simulink model "Drone_human_obstacle"  (R2024a)
settings: Solver=VariableStepAuto  StartTime=0.0  StopTime=10.0  RelTol=1e-3
undefined symbols (not defined in the file or in its folder): Angle, Axis, gray
libraries: eeGeneralControl x2, robotcorelib x1
settings Model: Creator=quentinlandon  LastModifiedBy=quentinlandon

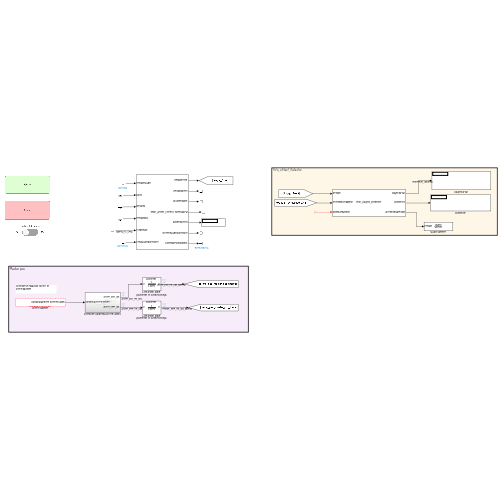
[thumbnail: Simulink's stored preview of the top-level diagram]
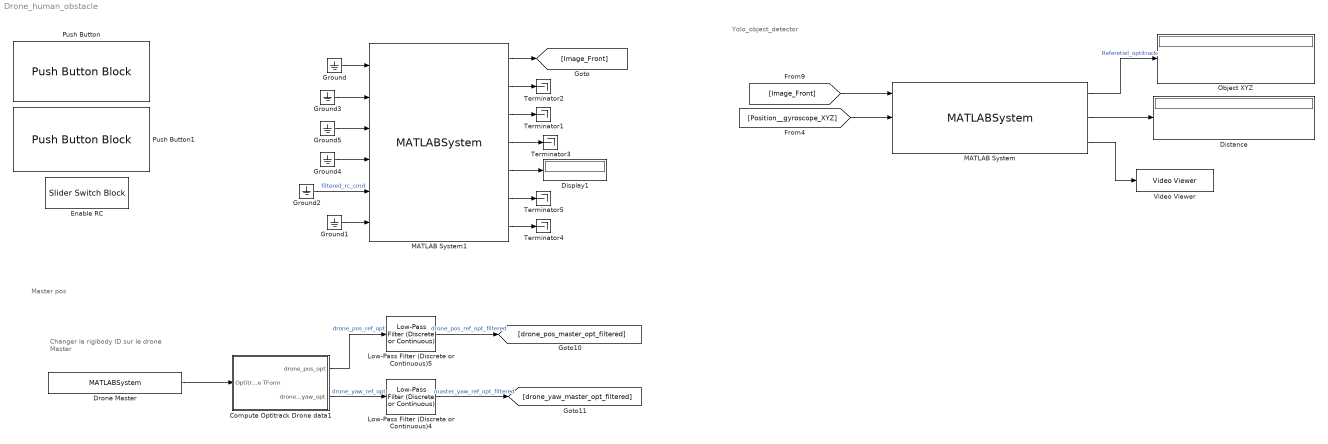
== system Drone_human_obstacle ==
  note: Changer le rigibody ID sur le drone Master
  note: Master pos
  note: Yolo_object_detector
  Compute Optitrack Drone data1 : Subsystem
  Display1 : Display
  Distance : Display
  Drone Master : MATLABSystem  System=OptilinkSystem  HostIP=10.147.125.15  ClientIP=10.147.125.15  RigidbodyID=1  SimulateUsing=Interpreted execution
      mask Type: OptilinkSystem
      mask Display:
      | disp('OptilinkSystem');
      | port_label('output',1,'Drones data');
  Enable RC : SliderSwitchBlock
      settings: Values={{'Off', 'On'}, [0 1]}
  Ground{,1..5} (6 alike) : Ground
  Low-Pass Filter (Discrete or Continuous)4 : eeGeneralControl/Low-Pass Filter (Discrete or Continuous)  K=1  T=1.5  B=inf  A=-inf  init_option=Inherited from block input  x0=0  Ts=-1
  Low-Pass Filter (Discrete or Continuous)5 : eeGeneralControl/Low-Pass Filter (Discrete or Continuous)  K=1  T=1.5  B=inf  A=-inf  init_option=Inherited from block input  x0=0  Ts=-1
  MATLAB System : MATLABSystem  System=Yolo_Object_Detector  SimulateUsing=Interpreted execution
      mask Type: Yolo_Object_Detector
      mask Display:
      | disp('Yolo_Object_Detector');
      | port_label('input',1,'Image');
      | port_label('input',2,'TranslationMatrix');
      | port_label('input',3,'RotationMatrix');
      | port_label('output',1,'ObjectXYZ');
      | port_label('output',2,'Distance');
      | port_label('output',3,'AnnotatedImage');
  MATLAB System1 : MATLABSystem  System=Tello_drone_control  droneIP=127.0.0.1  SimulateUsing=Interpreted execution
      mask Type: Tello_drone_control
      mask Display:
      | disp('Tello_drone_control');
      | port_label('input',1,'enableVideo');
      | port_label('input',2,'tkoff');
      | port_label('input',3,'landing');
      | port_label('input',4,'enableRC');
      | port_label('input',5,'rcspeeds');
      | port_label('input',6,'cmdVideoDirection');
      | port_label('output',1,'imageFront');
      | port_label('output',2,'imageDown');
      | port_label('output',3,'Eulerangles');
      | port_label('output',4,'speedXYZ');
      | port_label('output',5,'batteryLevel');
      | port_label('output',6,'currentVideoDirection');
      | port_label('output',7,'hasTakenOffStatus');
  Object XYZ : Display
  Push Button : PushButtonBlock  ButtonText=Décoler  OffValue=0.000000
  Push Button1 : PushButtonBlock  ButtonText=Atterir  OffValue=0.000000
  Terminator{1..5} (5 alike) : Terminator
  Video Viewer : VideoViewer  colormapValue=gray(256)  FigPos=[139 735 730 455]
  wires:
  Ground5/1 -> MATLAB System1/3
  MATLAB System1/6 -> Terminator5/1
  MATLAB System1/3 -> Terminator1/1
  Drone Master/1 -> Compute Optitrack Drone data1/1(Optitrack Drone TForm)
  Low-Pass Filter (Discrete or Continuous)4/1 -> [drone_yaw_master_opt_filtered]  "master_yaw_ref_opt_filtered"
  Ground3/1 -> MATLAB System1/2
  Ground2/1 -> MATLAB System1/5  "filtered_rc_cmd"
  Ground1/1 -> MATLAB System1/6
  Low-Pass Filter (Discrete or Continuous)5/1 -> [drone_pos_master_opt_filtered]  "drone_pos_ref_opt_filtered"
  Ground4/1 -> MATLAB System1/4
  Compute Optitrack Drone data1/2(drone_yaw_opt) -> Low-Pass Filter (Discrete or Continuous)4/1  "drone_yaw_ref_opt"
  MATLAB System1/7 -> Terminator4/1
  MATLAB System1/5 -> Display1/1
  MATLAB System1/1 -> [Image_Front]
  MATLAB System1/4 -> Terminator3/1
  Compute Optitrack Drone data1/1(drone_pos_opt) -> Low-Pass Filter (Discrete or Continuous)5/1  "drone_pos_ref_opt"
  Ground/1 -> MATLAB System1/1
  MATLAB System1/2 -> Terminator2/1
  ? -> MATLAB System/3
  [Image_Front] -> MATLAB System/1
  MATLAB System/2 -> Distance/1
  [Position__gyroscope_XYZ] -> MATLAB System/2
  MATLAB System/3 -> Video Viewer/1
  MATLAB System/1 -> Object XYZ/1  "Referetiel_optitrack"

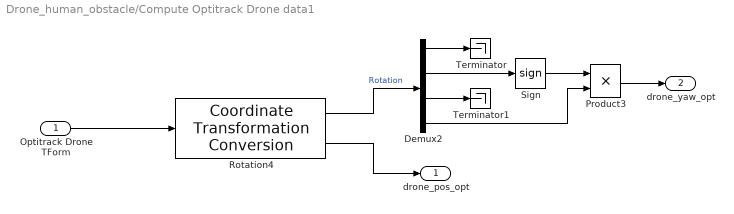
== system Drone_human_obstacle/Compute Optitrack Drone data1 ==
  Optitrack Drone TForm : Inport
  Demux2 : Demux
  Product3 : Product
  Rotation4 : robotcorelib/Coordinate Transformation Conversion  InputRepresentation=Homogeneous Transformation  InputEulerSequence=XYZ  ShowTrVecInputPort=on  OutputRepresentation=Axis-Angle  OutputEulerSequence=XYZ  ShowTrVecOutputPort=on  SimulateUsing=Code generation
      settings: LibrarySourceBlock=uavutilslib/Coordinate Transformation Conversion
  Sign : Signum
  Terminator : Terminator
  Terminator1 : Terminator
  drone_pos_opt : Outport
  drone_yaw_opt : Outport  Port=2
  wires:
  Rotation4/2 -> drone_pos_opt/1
  Demux2/4 -> Product3/2
  Rotation4/1 -> Demux2/1  "Rotation"
  Sign/1 -> Product3/1
  Demux2/2 -> Sign/1
  Product3/1 -> drone_yaw_opt/1
  Optitrack Drone TForm/1 -> Rotation4/1
  Demux2/3 -> Terminator1/1
  Demux2/1 -> Terminator/1
